simulink model "dsogi_pll_3ph"  (R2023a)
settings: Solver=FixedStepDiscrete  StartTime=0.0  StopTime=7/50  FixedStep=ts/40  RelTol=1e-3
InitFcn:
  | ts=1/10e3;
  | volts=230*sqrt(2)*3.3/700;
  | freq=2*pi*50;
  | phase=pi;
  | 
  | wn_pi=80*2*pi;%200*2*pi;
  | sig_pi=.07;%.05;
  | vac_peak_pi=230*sqrt(2)*3.3/350;
  | kp =2*wn_pi*sig_pi/vac_peak_pi;
  | ki = vac_peak_pi/(4*sig_pi*sig_pi);
  | sig=2.5;
  | wn=2*pi*100;
  | Kg=1.2;
  | 
  | phsw_marg=.1;
  | ts_phsw=1/66;
libraries: eeGeneralControl x1
settings Model: DataDictionary=dictionary.sldd  MinMaxOverflowLogging=MinMaxAndOverflow  FPTRunName=BaselineRun  Creator=ASUSTUF  LastModifiedBy=ASUSTUF
settings OptimizationCC: DefaultParameterBehavior=Inlined  UseDivisionForNetSlopeComputation=on  GainParamInheritBuiltInType=on  UseFloatMulNetSlope=on  InlineInvariantSignals=on  EnhancedBackFolding=on  PassReuseOutputArgsAs=Individual arguments  ZeroExternalMemoryAtStartup=off  ZeroInternalMemoryAtStartup=off  EfficientFloat2IntCast=on  OptimizeBlockOrder=speed  DifferentSizesBufferReuse=on  OptimizationCustomize=off  EfficientTunableParamExpr=on
settings DebuggingCC: SignalRangeChecking=warning  ParameterTunabilityLossMsg=error
settings HardwareCC: ProdLongLongMode=on
settings SFSimCC: MATLABDynamicMemAlloc=off
settings RTWCC: Description=Embedded Coder  SystemTargetFile=ert.tlc  TemplateMakefile=ert_default_tmf  GenerateReport=on  LaunchReport=on
settings CodeAppCC: ForceParamTrailComments=on  IgnoreCustomStorageClasses=off  OperatorAnnotations=on  SimulinkDataObjDesc=on  SFDataObjDesc=on  InsertBlockDesc=on
settings ERTTargetCC: TargetLangStandard=C99 (ISO)  GenerateSampleERTMain=on  InlinedParameterPlacement=NonHierarchical  ERTCustomFileTemplate=example_file_process.tlc

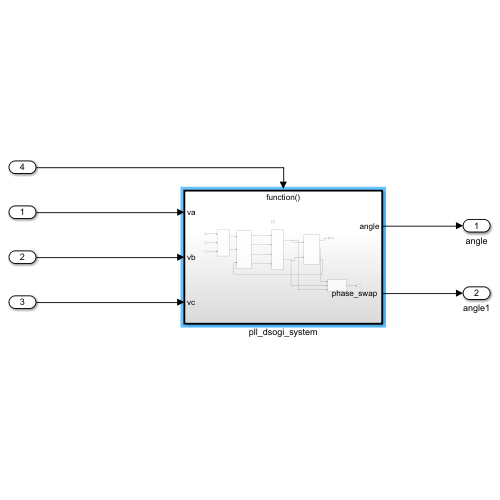
[thumbnail: Simulink's stored preview of the top-level diagram]
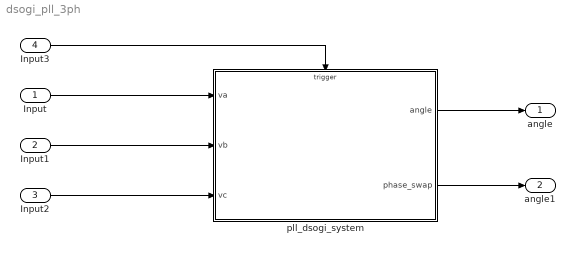
== system dsogi_pll_3ph ==
  Input : Inport
  Input1 : Inport  Port=2
  Input2 : Inport  Port=3
  Input3 : Inport  Port=4  SampleTime=ts  OutputFunctionCall=on
  pll_dsogi_system : Subsystem  TreatAsAtomicUnit=on
  angle : Outport
  angle1 : Outport  Port=2
  wires:
  Input/1 -> pll_dsogi_system/1(va)
  Input1/1 -> pll_dsogi_system/2(vb)
  Input2/1 -> pll_dsogi_system/3(vc)
  Input3/1 -> pll_dsogi_system/Trigger
  pll_dsogi_system/1(angle) -> angle/1
  pll_dsogi_system/2("phase_swap ") -> angle1/1

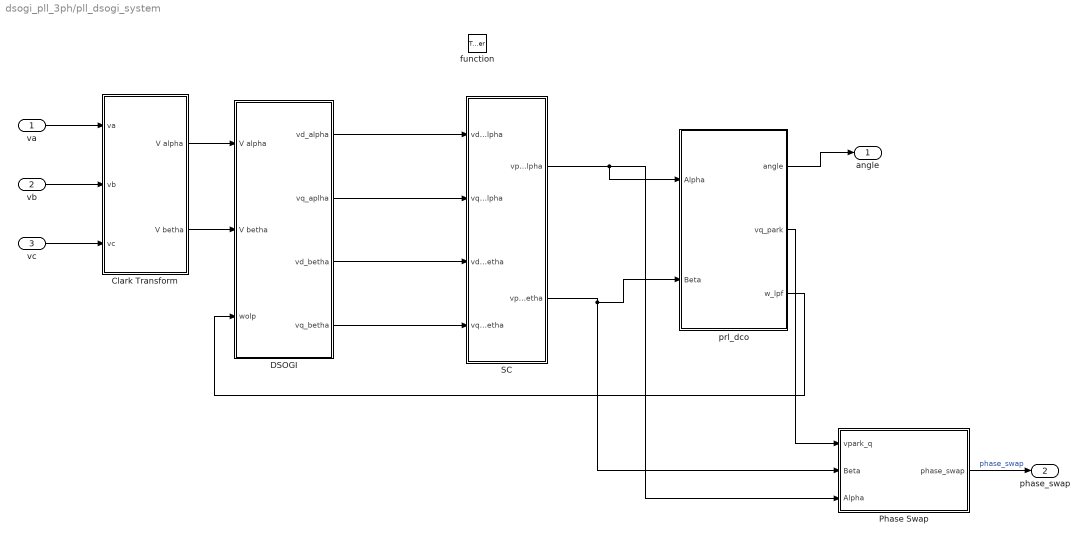
== system dsogi_pll_3ph/pll_dsogi_system ==
  va : Inport  OutDataTypeStr=double
  vb : Inport  Port=2  OutDataTypeStr=double
  vc : Inport  Port=3  OutDataTypeStr=double
  function : TriggerPort  TriggerType=function-call  VariantControl=(inherit)
  Clark Transform : Subsystem  SystemSampleTime=ts
  DSOGI : Subsystem  SystemSampleTime=ts
  Phase Swap : Subsystem
  SC : Subsystem  SystemSampleTime=ts
  prl_dco : Subsystem
  angle : Outport
  "phase_swap " : Outport  Port=2
  wires:
  prl_dco/1(angle) -> angle/1
  SC/2(vp_betha) -> prl_dco/2(Beta), Phase Swap/2(Beta)
  DSOGI/4(vq_betha) -> SC/4(vq_sogi_betha)
  vc/1 -> Clark Transform/3(vc)
  DSOGI/3(vd_betha) -> SC/3(vd_sogi_betha)
  va/1 -> Clark Transform/1(va)
  SC/1(vp_alpha) -> prl_dco/1(Alpha), Phase Swap/3(Alpha)
  Clark Transform/2(V betha) -> DSOGI/2(V betha)
  vb/1 -> Clark Transform/2(vb)
  Clark Transform/1(V alpha) -> DSOGI/1(V alpha)
  DSOGI/1(vd_alpha) -> SC/1(vd_sogi_alpha)
  prl_dco/3(w_lpf) -> DSOGI/3(wolp)
  DSOGI/2(vq_aplha) -> SC/2(vq_sogi_alpha)
  Phase Swap/1("phase_swap ") -> "phase_swap "/1  "phase_swap"
  prl_dco/2(vq_park) -> Phase Swap/1(vpark_q)

== system dsogi_pll_3ph/pll_dsogi_system/Clark Transform ==
  va : Inport  OutDataTypeStr=double
  vb : Inport  Port=2  OutDataTypeStr=double
  vc : Inport  Port=3  OutDataTypeStr=double
  clark_trafo : MATLAB Function  TreatAsAtomicUnit=on
  V alpha : Outport
  V betha : Outport  Port=2
  wires:
  va/1 -> clark_trafo/1(va)
  vb/1 -> clark_trafo/2(vb)
  vc/1 -> clark_trafo/3(vc)
  clark_trafo/1(valpha) -> V alpha/1  "V alpha"
  clark_trafo/2(vbetha) -> V betha/1  "V betha"

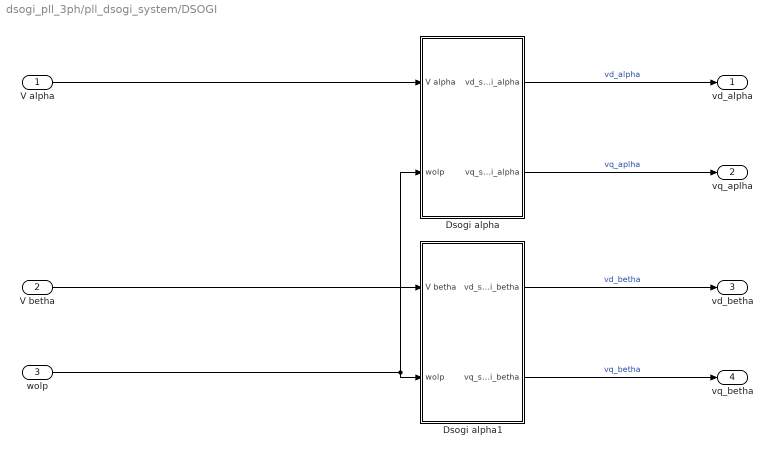
== system dsogi_pll_3ph/pll_dsogi_system/DSOGI ==
  V alpha : Inport  OutDataTypeStr=double
  V betha : Inport  Port=2  OutDataTypeStr=double
  wolp : Inport  Port=3  OutDataTypeStr=double
  Dsogi alpha : Subsystem
  Dsogi alpha1 : Subsystem
  vd_alpha : Outport
  vq_aplha : Outport  Port=2
  vd_betha : Outport  Port=3
  vq_betha : Outport  Port=4
  wires:
  Dsogi alpha/2(vq_sogi_alpha) -> vq_aplha/1  "vq_aplha"
  Dsogi alpha1/1(vd_sogi_betha) -> vd_betha/1  "vd_betha"
  wolp/1 -> Dsogi alpha1/2(wolp), Dsogi alpha/2(wolp)
  V betha/1 -> Dsogi alpha1/1(V betha)
  Dsogi alpha1/2(vq_sogi_betha) -> vq_betha/1  "vq_betha"
  V alpha/1 -> Dsogi alpha/1(V alpha)
  Dsogi alpha/1(vd_sogi_alpha) -> vd_alpha/1  "vd_alpha"

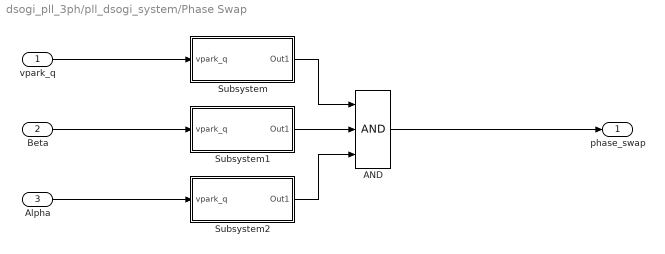
== system dsogi_pll_3ph/pll_dsogi_system/Phase Swap ==
  vpark_q : Inport  OutDataTypeStr=double
  Beta : Inport  Port=2  OutDataTypeStr=double
  Alpha : Inport  Port=3  OutDataTypeStr=double
  AND : Logic  Inputs=3  IconShape=distinctive  AllPortsSameDT=off  OutDataTypeStr=boolean
  Subsystem : Subsystem
  Subsystem1 : Subsystem
  Subsystem2 : Subsystem
  "phase_swap " : Outport
  wires:
  Subsystem/1(Out1) -> AND/1
  Subsystem1/1(Out1) -> AND/2
  Subsystem2/1(Out1) -> AND/3
  Beta/1 -> Subsystem1/1(vpark_q)
  Alpha/1 -> Subsystem2/1(vpark_q)
  vpark_q/1 -> Subsystem/1(vpark_q)
  AND/1 -> "phase_swap "/1

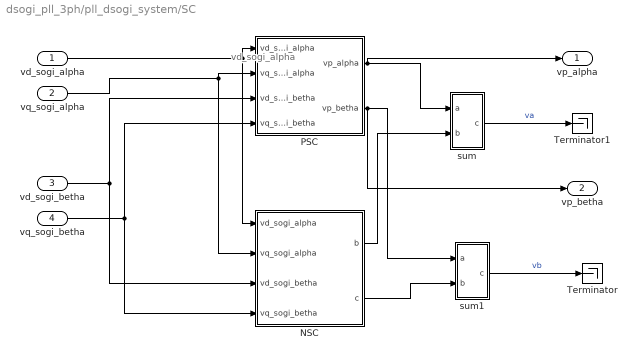
== system dsogi_pll_3ph/pll_dsogi_system/SC ==
  note: vd_sogi_alpha
  vd_sogi_alpha : Inport  OutDataTypeStr=double
  vq_sogi_alpha : Inport  Port=2  OutDataTypeStr=double
  vd_sogi_betha : Inport  Port=3  OutDataTypeStr=double
  vq_sogi_betha : Inport  Port=4  OutDataTypeStr=double
  NSC : Subsystem
  PSC : Subsystem
  Terminator : Terminator
  Terminator1 : Terminator
  sum : MATLAB Function  TreatAsAtomicUnit=on  VariantControl=false()
  sum1 : MATLAB Function  TreatAsAtomicUnit=on  VariantControl=false()
  vp_alpha : Outport
  vp_betha : Outport  Port=2
  wires:
  vd_sogi_alpha/1 -> NSC/1(vd_sogi_alpha), PSC/1(vd_sogi_alpha)
  vq_sogi_alpha/1 -> PSC/2(vq_sogi_alpha), NSC/2(vq_sogi_alpha)
  vd_sogi_betha/1 -> NSC/3(vd_sogi_betha), PSC/3(vd_sogi_betha)
  vq_sogi_betha/1 -> NSC/4(vq_sogi_betha), PSC/4(vq_sogi_betha)
  PSC/1(vp_alpha) -> sum/1(a), vp_alpha/1
  PSC/2(vp_betha) -> sum1/1(a), vp_betha/1
  NSC/1(b) -> sum/2(b)
  sum/1(c) -> Terminator1/1  "va"
  NSC/2(c) -> sum1/2(b)
  sum1/1(c) -> Terminator/1  "vb"

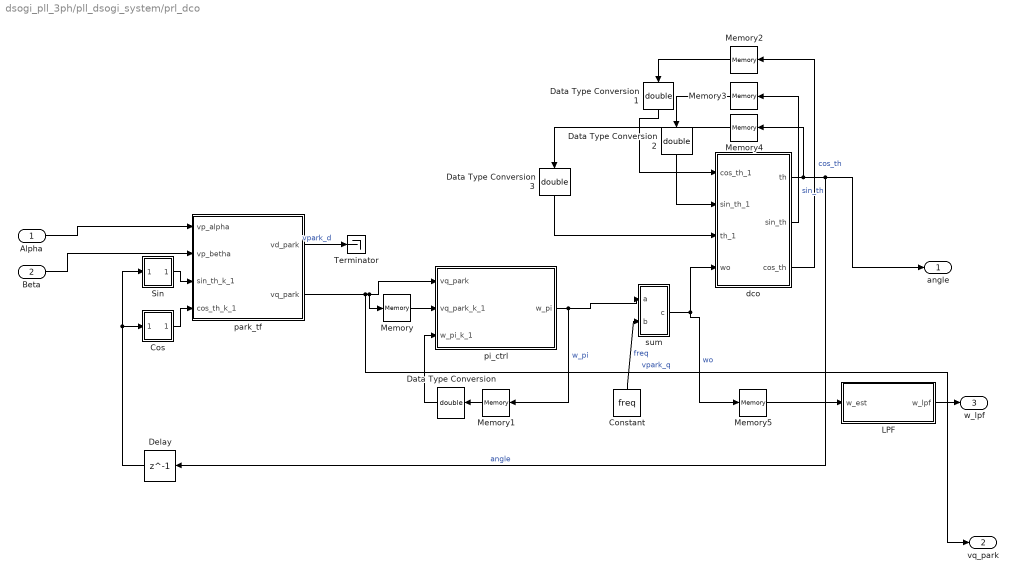
== system dsogi_pll_3ph/pll_dsogi_system/prl_dco ==
  Alpha : Inport  OutDataTypeStr=double
  Beta : Inport  Port=2  OutDataTypeStr=double
  Constant : Constant  Value=freq  OutDataTypeStr=double
  Cos : Subsystem  Tag=DecoupledSystem
  Data Type Conversion{,1..3} (4 alike) : DataTypeConversion  OutDataTypeStr=double  SaturateOnIntegerOverflow=off  RndMeth=Floor
  Delay : Delay  DelayLength=1
  LPF : Subsystem
  Memory{,1,3..4} (4 alike) : Memory  InheritSampleTime=on
  Memory2 : Memory  InitialCondition=.99  InheritSampleTime=on
  Memory5 : Memory  InitialCondition=freq  InheritSampleTime=on
  Sin : Subsystem  Tag=DecoupledSystem
  Terminator : Terminator
  dco : MATLAB Function  TreatAsAtomicUnit=on  VariantControl=false()
  park_tf : MATLAB Function  TreatAsAtomicUnit=on  VariantControl=false()
  pi_ctrl : MATLAB Function  TreatAsAtomicUnit=on  VariantControl=false()
  sum : MATLAB Function  TreatAsAtomicUnit=on  VariantControl=false()
  angle : Outport
  vq_park : Outport  Port=2
  w_lpf : Outport  Port=3
  wires:
  Memory1/1 -> Data Type Conversion/1
  Data Type Conversion2/1 -> dco/2(sin_th_1)
  Memory5/1 -> LPF/1(w_est)
  Data Type Conversion/1 -> pi_ctrl/3(w_pi_k_1)
  dco/1(th) -> angle/1, Delay/1, Memory4/1  "angle"
  Memory2/1 -> Data Type Conversion1/1
  Beta/1 -> park_tf/2(vp_betha)
  Alpha/1 -> park_tf/1(vp_alpha)
  Memory4/1 -> Data Type Conversion3/1
  dco/3(cos_th) -> Memory2/1  "cos_th"
  park_tf/2(vq_park) -> vq_park/1, pi_ctrl/1(vq_park), Memory/1  "vpark_q"
  Memory/1 -> pi_ctrl/2(vq_park_k_1)
  dco/2(sin_th) -> Memory3/1  "sin_th"
  park_tf/1(vd_park) -> Terminator/1  "vpark_d"
  Sin/1(Out1) -> park_tf/3(sin_th_k_1)
  Data Type Conversion3/1 -> dco/3(th_1)
  LPF/1(w_lpf) -> w_lpf/1
  sum/1(c) -> dco/4(wo), Memory5/1  "wo"
  Delay/1 -> Sin/1(In1), Cos/1(In1)
  Cos/1(Out1) -> park_tf/4(cos_th_k_1)
  pi_ctrl/1(w_pi) -> sum/1(a), Memory1/1  "w_pi"
  Data Type Conversion1/1 -> dco/1(cos_th_1)
  Memory3/1 -> Data Type Conversion2/1
  Constant/1 -> sum/2(b)  "freq"

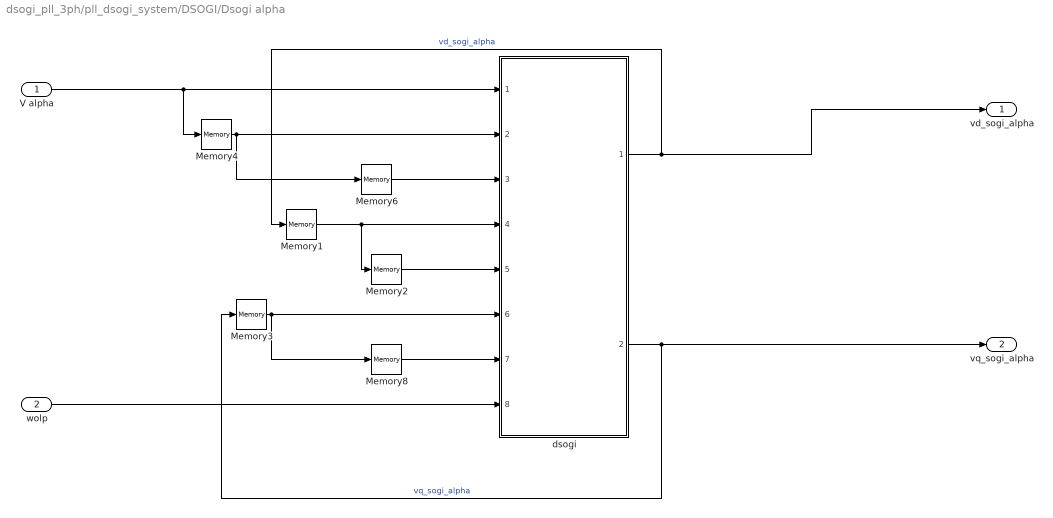
== system dsogi_pll_3ph/pll_dsogi_system/DSOGI/Dsogi alpha ==
  V alpha : Inport  OutMin=[-1.6]  OutMax=[1.6]  OutDataTypeStr=double
  wolp : Inport  Port=2  OutMin=[2*pi*45]  OutMax=[2*pi*65]  OutDataTypeStr=double
  Memory{1..4,6,8} (6 alike) : Memory  InheritSampleTime=on
  dsogi : Subsystem  ReferencedSubsystem=dsogi
  vd_sogi_alpha : Outport  OutMin=[-1.6]  OutMax=[1.6]
  vq_sogi_alpha : Outport  Port=2  OutMin=[-1.6]  OutMax=[1.6]
  wires:
  V alpha/1 -> dsogi/1, Memory4/1
  Memory4/1 -> dsogi/2, Memory6/1
  Memory1/1 -> dsogi/4, Memory2/1
  Memory3/1 -> dsogi/6, Memory8/1
  Memory6/1 -> dsogi/3
  Memory2/1 -> dsogi/5
  Memory8/1 -> dsogi/7
  wolp/1 -> dsogi/8
  dsogi/1 -> vd_sogi_alpha/1, Memory1/1  "vd_sogi_alpha"
  dsogi/2 -> vq_sogi_alpha/1, Memory3/1  "vq_sogi_alpha"

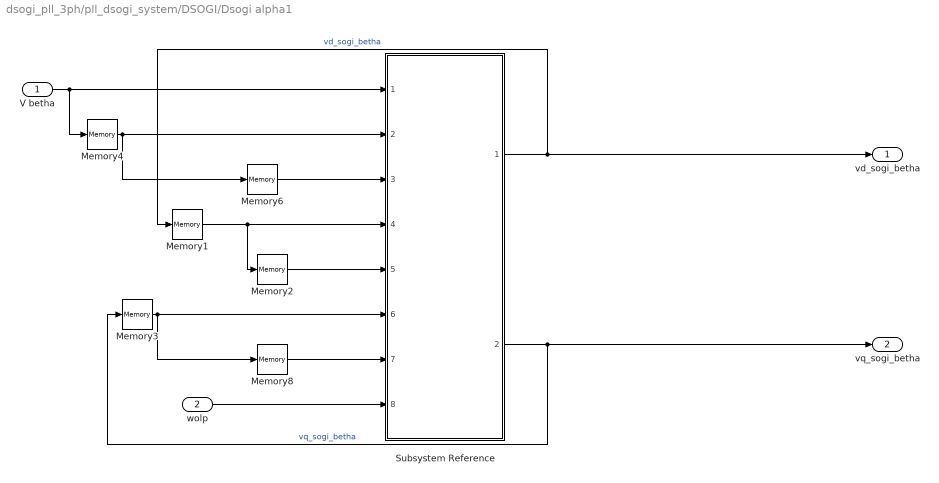
== system dsogi_pll_3ph/pll_dsogi_system/DSOGI/Dsogi alpha1 ==
  V betha : Inport  OutMin=[-1.6]  OutMax=[1.6]  OutDataTypeStr=double
  wolp : Inport  Port=2  OutMin=[2*pi*45]  OutMax=[2*pi*65]  OutDataTypeStr=double
  Memory{1..4,6,8} (6 alike) : Memory  InheritSampleTime=on
  Subsystem Reference : Subsystem  ReferencedSubsystem=dsogi
  vd_sogi_betha : Outport  OutMin=[-1.6]  OutMax=[1.6]
  vq_sogi_betha : Outport  Port=2  OutMin=[-1.6]  OutMax=[1.6]
  wires:
  Memory3/1 -> Subsystem Reference/6, Memory8/1
  Memory1/1 -> Subsystem Reference/4, Memory2/1
  Memory4/1 -> Subsystem Reference/2, Memory6/1
  V betha/1 -> Subsystem Reference/1, Memory4/1
  Memory6/1 -> Subsystem Reference/3
  Memory2/1 -> Subsystem Reference/5
  Memory8/1 -> Subsystem Reference/7
  wolp/1 -> Subsystem Reference/8
  Subsystem Reference/1 -> vd_sogi_betha/1, Memory1/1  "vd_sogi_betha"
  Subsystem Reference/2 -> Memory3/1, vq_sogi_betha/1  "vq_sogi_betha"

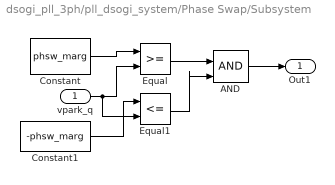
== system dsogi_pll_3ph/pll_dsogi_system/Phase Swap/Subsystem ==
  vpark_q : Inport  OutDataTypeStr=double
  AND : Logic  IconShape=distinctive  AllPortsSameDT=off  OutDataTypeStr=boolean
  Constant : Constant  Value=phsw_marg  OutDataTypeStr=double
  Constant1 : Constant  Value=-phsw_marg  OutDataTypeStr=double
  Equal : RelationalOperator  OutDataTypeStr=boolean  RndMeth=Simplest  InputSameDT=off
  Equal1 : RelationalOperator  Operator=<=  OutDataTypeStr=boolean  RndMeth=Simplest  InputSameDT=off
  Out1 : Outport
  wires:
  Constant/1 -> Equal/1
  vpark_q/1 -> Equal1/2, Equal/2
  Equal/1 -> AND/1
  Equal1/1 -> AND/2
  AND/1 -> Out1/1
  Constant1/1 -> Equal1/1

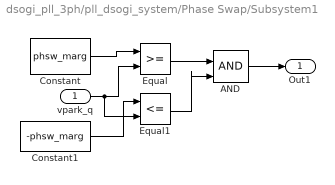
== system dsogi_pll_3ph/pll_dsogi_system/Phase Swap/Subsystem1 ==
  vpark_q : Inport  OutDataTypeStr=double
  AND : Logic  IconShape=distinctive  AllPortsSameDT=off  OutDataTypeStr=boolean
  Constant : Constant  Value=phsw_marg  OutDataTypeStr=double
  Constant1 : Constant  Value=-phsw_marg  OutDataTypeStr=double
  Equal : RelationalOperator  OutDataTypeStr=boolean  RndMeth=Simplest  InputSameDT=off
  Equal1 : RelationalOperator  Operator=<=  OutDataTypeStr=boolean  RndMeth=Simplest  InputSameDT=off
  Out1 : Outport
  wires:
  Constant1/1 -> Equal1/1
  AND/1 -> Out1/1
  Equal1/1 -> AND/2
  Equal/1 -> AND/1
  vpark_q/1 -> Equal/2, Equal1/2
  Constant/1 -> Equal/1

== system dsogi_pll_3ph/pll_dsogi_system/Phase Swap/Subsystem2 ==
  vpark_q : Inport  OutDataTypeStr=double
  AND : Logic  IconShape=distinctive  AllPortsSameDT=off  OutDataTypeStr=boolean
  Constant : Constant  Value=phsw_marg  OutDataTypeStr=double
  Constant1 : Constant  Value=-phsw_marg  OutDataTypeStr=double
  Equal : RelationalOperator  OutDataTypeStr=boolean  RndMeth=Simplest  InputSameDT=off
  Equal1 : RelationalOperator  Operator=<=  OutDataTypeStr=boolean  RndMeth=Simplest  InputSameDT=off
  Out1 : Outport
  wires:
  Constant/1 -> Equal/1
  vpark_q/1 -> Equal1/2, Equal/2
  Equal/1 -> AND/1
  Equal1/1 -> AND/2
  AND/1 -> Out1/1
  Constant1/1 -> Equal1/1

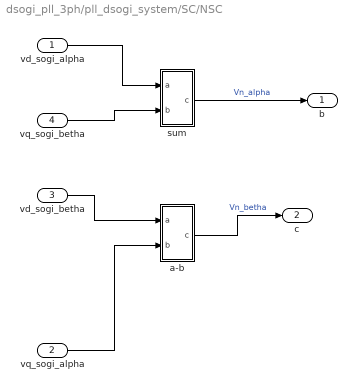
== system dsogi_pll_3ph/pll_dsogi_system/SC/NSC ==
  vd_sogi_alpha : Inport  OutDataTypeStr=double
  vq_sogi_alpha : Inport  Port=2  OutDataTypeStr=double
  vd_sogi_betha : Inport  Port=3  OutDataTypeStr=double
  vq_sogi_betha : Inport  Port=4  OutDataTypeStr=double
  a-b : MATLAB Function  TreatAsAtomicUnit=on  VariantControl=false()
  sum : MATLAB Function  TreatAsAtomicUnit=on  VariantControl=false()
  b : Outport
  c : Outport  Port=2
  wires:
  vd_sogi_betha/1 -> a-b/1(a)
  vq_sogi_alpha/1 -> a-b/2(b)
  a-b/1(c) -> c/1  "Vn_betha"
  vd_sogi_alpha/1 -> sum/1(a)
  vq_sogi_betha/1 -> sum/2(b)
  sum/1(c) -> b/1  "Vn_alpha"

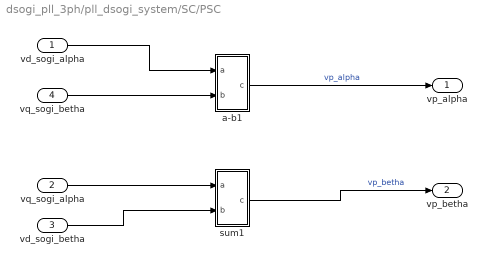
== system dsogi_pll_3ph/pll_dsogi_system/SC/PSC ==
  vd_sogi_alpha : Inport  OutDataTypeStr=double
  vq_sogi_alpha : Inport  Port=2  OutDataTypeStr=double
  vd_sogi_betha : Inport  Port=3  OutDataTypeStr=double
  vq_sogi_betha : Inport  Port=4  OutDataTypeStr=double
  a-b1 : MATLAB Function  TreatAsAtomicUnit=on  VariantControl=false()
  sum1 : MATLAB Function  TreatAsAtomicUnit=on  VariantControl=false()
  vp_alpha : Outport
  vp_betha : Outport  Port=2
  wires:
  vq_sogi_alpha/1 -> sum1/1(a)
  vd_sogi_betha/1 -> sum1/2(b)
  sum1/1(c) -> vp_betha/1  "vp_betha"
  vd_sogi_alpha/1 -> a-b1/1(a)
  vq_sogi_betha/1 -> a-b1/2(b)
  a-b1/1(c) -> vp_alpha/1  "vp_alpha"

== system dsogi_pll_3ph/pll_dsogi_system/prl_dco/Cos ==
  In1 : Inport  LockScale=on
  ReplicaOfSource : Trigonometry  Operator=cos
  Out1 : Outport  LockScale=on
  wires:
  ReplicaOfSource/1 -> Out1/1
  In1/1 -> ReplicaOfSource/1

== system dsogi_pll_3ph/pll_dsogi_system/prl_dco/LPF ==
  w_est : Inport  OutDataTypeStr=double
  Low-Pass Filter (Discrete or Continuous) : Subsystem  Tag=DecoupledSystem
  w_lpf : Outport
  wires:
  w_est/1 -> Low-Pass Filter (Discrete or Continuous)/1(In1)
  Low-Pass Filter (Discrete or Continuous)/1(Out1) -> w_lpf/1  "w_lpf"

== system dsogi_pll_3ph/pll_dsogi_system/prl_dco/Sin ==
  In1 : Inport  LockScale=on
  ReplicaOfSource : Trigonometry
  Out1 : Outport  LockScale=on
  wires:
  ReplicaOfSource/1 -> Out1/1
  In1/1 -> ReplicaOfSource/1

== system dsogi_pll_3ph/pll_dsogi_system/prl_dco/LPF/Low-Pass Filter (Discrete or Continuous) ==
  In1 : Inport  LockScale=on
  ReplicaOfSource : eeGeneralControl/Low-Pass Filter (Discrete or Continuous)  K=1  T=1/7e2  B=inf  A=-inf  init_option=Inherited from block input  x0=0  Ts=-1
  Out1 : Outport  LockScale=on
  wires:
  ReplicaOfSource/1 -> Out1/1
  In1/1 -> ReplicaOfSource/1

== matlab function dsogi_pll_3ph/pll_dsogi_system/prl_dco/sum ==
  data: a input; c output; b input
function c = fcn(a,b)

c=a+b;
end

== matlab function dsogi_pll_3ph/pll_dsogi_system/Clark Transform/clark_trafo ==
  data: va input; valpha output; vb input; vc input; vbetha output
function [valpha, vbetha] = clarktrans(va,vb,vc)
fimath('RoundingMethod', 'Floor', ...
'OverflowAction', 'Saturate', ...
'ProductMode', 'SpecifyPrecision', ...
'ProductWordLength', 16, ...
'ProductFractionLength', 2, ...
'SumMode', 'SpecifyPrecision', ...
'SumWordLength', 16, ...
'SumFractionLength', 2, ...
'CastBeforeSum', true)

valpha=((2/3)*(va-(.5*vb)-(.5*vc)));
vbetha=( ((2/3)*(sqrt(3)*.5))*(vb-vc) );

end

== matlab function dsogi_pll_3ph/pll_dsogi_system/SC/NSC/a-b ==
  data: a input; c output; b input
function c = fcn(a,b)

c=0.5*(a-b);
end

== matlab function dsogi_pll_3ph/pll_dsogi_system/SC/NSC/sum ==
  data: a input; c output; b input
function c = fcn(a,b)

c=0.5*(a+b);
end

== matlab function dsogi_pll_3ph/pll_dsogi_system/SC/PSC/a-b1 ==
  data: a input; c output; b input
function c = fcn(a,b)

c=0.5*(a-b);
end

== matlab function dsogi_pll_3ph/pll_dsogi_system/SC/PSC/sum1 ==
  data: a input; c output; b input
function c = fcn(a,b)

c=0.5*(a+b);
end

== matlab function dsogi_pll_3ph/pll_dsogi_system/SC/sum ==
  data: a input; c output; b input
function c = fcn(a,b)

c=(a-b);
end

== matlab function dsogi_pll_3ph/pll_dsogi_system/SC/sum1 ==
  data: a input; c output; b input
function c = fcn(a,b)

c=(a-b);
end

== matlab function dsogi_pll_3ph/pll_dsogi_system/prl_dco/dco ==
  data: cos_th_1 input; sin_th_1 input; th_1 input; th output; sin_th output; wo input; cos_th output
function [th,sin_th,cos_th]= dco(cos_th_1,sin_th_1,th_1,wo)
        % ws=(2*pi*50);
        wout=(wo);
        tsample=1/10e3;
        %Sin is for showing the overlaping w the input 
        sin_th=sin_th_1+(cos_th_1*wout*tsample);%Sin(t+dt)=sin(t)+cos(t)*dt
        cos_th=cos_th_1-(sin_th_1*wout*tsample);
        
        sin_th=max([sin_th -1]);
        cos_th=max([cos_th -1]);

        sin_th=min([sin_th 1]);
        cos_th=min([cos_th 1]);

        th=th_1+(wout*tsample);

        if sin_th_1>=0 && sin_th<=0
            th=-pi;%fi(pi,1,32,29); %zero crossing reseting phase angle
        end
      
end

== matlab function dsogi_pll_3ph/pll_dsogi_system/prl_dco/park_tf ==
  data: vd_park output; vp_alpha input; vq_park output; vp_betha input; sin_th_k_1 input; cos_th_k_1 input
function [vd_park,vq_park] = park(vp_alpha,vp_betha,sin_th_k_1,cos_th_k_1)

vq_park=(sin_th_k_1*vp_betha+cos_th_k_1*vp_alpha);%(-sin_th_k_1*vp_alpha+cos_th_k_1*vp_betha);
vd_park=(sin_th_k_1*vp_alpha-cos_th_k_1*vp_betha);




end

== matlab function dsogi_pll_3ph/pll_dsogi_system/prl_dco/pi_ctrl ==
  data: vq_park input; w_pi output; vq_park_k_1 input; w_pi_k_1 input
function w_pi = pi_ctrl(vq_park,vq_park_k_1,w_pi_k_1)

fs=10e3;ts=1/fs;
wn_pi=100*2*pi;%200*2*pi; 
sig_pi=.5;%.05;
vac_peak_pi=.3*3.3;

kp =2*wn_pi*sig_pi/vac_peak_pi;
ki = vac_peak_pi/(4*sig_pi*sig_pi);

pi_n1=kp;
pi_n2=(ki*ts)-kp;


w_pi=((vq_park)*pi_n1+(vq_park_k_1)*pi_n2+w_pi_k_1);

end
